simulink library "environment_cl"  (R2018a)
settings: Solver=VariableStepAuto  StartTime=0.0  StopTime=10.0  RelTol=1e-3
libraries: cosineSquaredEnvr_ul x1
settings Model: Creator=mcobb  LastModifiedBy=mcobb

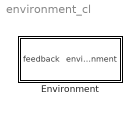
== system environment_cl ==
  Environment : Subsystem

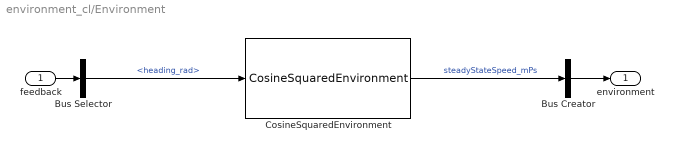
== system environment_cl/Environment ==
  feedback : Inport
  Bus Creator : BusCreator  Inputs=1
  Bus Selector : BusSelector  OutputSignals=heading_rad
  CosineSquaredEnvironment : cosineSquaredEnvr_ul/CosineSquaredEnvironment
  environment : Outport
  wires:
  feedback/1 -> Bus Selector/1
  CosineSquaredEnvironment/1 -> Bus Creator/1  "steadyStateSpeed_mPs"
  Bus Creator/1 -> environment/1
  Bus Selector/1 -> CosineSquaredEnvironment/1  "<heading_rad>"
